simulink model "ltao_e2e"  (R2022b)
settings: Solver=FixedStepDiscrete  StartTime=0.0  StopTime=30  FixedStep=FEM_Ts  MaxStep=FEM_Ts  RelTol=1e-2
InitFcn:
  | %
  | % Initialization callback function
  | %
  | 
  | try
  |    fprintf('\nGMT IMS version (%s)!\n',simulink_fname );
  | 
  |    % Get Simulink model directory
  |    [filepath,name,ext] = fileparts(which(bdroot));
  | 
  |    if ~strcmp(filepath,pwd)
  |       fprintf('\nChanging current directory to \n %s \n',filepath);
  |       cd(filepath);
  |    end
  | 
  |    %
  |  if(osim.bpless_wl)
  |     fprintf('Generating bumpless wind load time series\n');
  |  end
  | catch
  |    warning('Running the InitFcn from puSimulate script');
  | end
values from neighbouring files (symbols this model uses):
  asm_kl_dist = 0*asm_kl_dist    [load_ltao_e2e.m]
  asm_ssG = XiKL' * asm_ssG * XiKL    [load_ltao_e2e.m]
  Cpi_d = eye(n_Zmodes)* c2d(st.asm.fpi, Ts, c2d_opts)    [evalM2asm_modal.m]    (also in load_ltao_e2e.m = c2d(st.asm.fpi, FEM_Ts, c2d_opts))
  fao_d = c2d(st.glao.fao, st.glao.T, c2d_opts)    [evalM2asm_modal.m]    (also in load_ltao_e2e.m = c2d(st.ltao.fao, FEM_Ts, c2d_opts))
  fao_d4k = c2d(st.ltao.fao, 1/4e3, c2d_opts)    [evalM2asm_modal.m]    (also in load_ltao_e2e.m = c2d(st.ltao.fao, FEM_Ts, c2d_opts))
  FEM_Ts = 1/8e3    (= 0.000125)    [load_ltao_e2e.m]
  fes = c2d(tf((fc_es^2)*4*(pi^2),[1, 2*0.8*fc_es*2*pi, (fc_es^2)*4*(pi^2)]),     st.ltao.T,c2d_opts)    [load_ltao_e2e.m]
  flag_1stOdyn_d = tf(c2d(flag(2,1), Ts, c2d_opts))    [evalM2asm_modal.m]    (also in load_ltao_e2e.m = tf(c2d(flag(2,1),FEM_Ts,c2d_opts)))
  flag_2ndOdyn_d = tf(c2d(flag(3,1), Ts, c2d_opts))    [evalM2asm_modal.m]    (also in load_ltao_e2e.m = tf(c2d(flag(3,1),FEM_Ts,c2d_opts)))
  fm2off = c2d(f_ct_m2off, st.ltao.T,c2d_opts)    [load_ltao_e2e.m]
  fpre_d = tf(c2d(st.asm.fpre, Ts, c2d_opts))    [evalM2asm_modal.m]    (also in load_ltao_e2e.m = tf(c2d(fpre,FEM_Ts,c2d_opts)))
  gtt2mnt = eye(2)/(rbm2gtt * Hk_mnt_m1m2)    [load_ltao_e2e.m]
  Hk_mnt_m1m2 = Cm1m2*pinv(Cmnt)    [load_ltao_e2e.m]
  Hpd_d = eye(n_Zmodes)* c2d(st.asm.fpd, Ts, c2d_opts)    [evalM2asm_modal.m]    (also in load_ltao_e2e.m = c2d(st.asm.fpd, FEM_Ts, 'Tustin'))
  K_asm_2_m2p = K_m2p / K_m2p6F_2_asmRB    [load_ltao_e2e.m]
  K_m2p = gainMatrix(out_m2p_mc,in_m2p_mc) -gainMatrix(out_m2p_mc,in_m2p_m2)          - gainMatrix(out_m2p_m2,in_m2p_mc) +gainMatrix(out_m2p_m2,in_m2p_m2)    [load_ltao_e2e.m]
  K_m2p6F_2_asmRB = gainMatrix(out_asm_RB,in_m2p_mc) - gainMatrix(out_asm_RB,in_m2p_m2)    [load_ltao_e2e.m]
  K_m2p_2_asm = K_m2p6F_2_asmRB/ K_m2p    [load_ltao_e2e.m]
  K_m2p_2_es = gainMatrix(out_m2es,in_m2p_mc)-gainMatrix(out_m2es,in_m2p_m2)    [load_ltao_e2e.m]
  Kasmoff = K_asm_2_m2p *         [Kasmoff_{1},Kasmoff_{2},Kasmoff_{3},Kasmoff_{4},         Kasmoff_{5},Kasmoff_{6},Kasmoff_{7}]    [load_ltao_e2e.m]
  Ki_m2off = 1.3    [load_ltao_e2e.m]
  Km1rbm_es = (KhpF2es/KhpF2m1rbm)    [load_ltao_e2e.m]
  Ks = cell(7,1)    [load_ltao_e2e.m]
  m1_rbm_dist = zeros(42,1)    [load_ltao_e2e.m]
  m2_rbm_dist = 0*m2_rbm_dist    [load_ltao_e2e.m]
  m2_rbm_offset = 0*m2_rbm_offset    [load_ltao_e2e.m]
  PG = zeros(length(om2),6)    [evalM2asm_modal.m]    (also in load_ltao_e2e.m)
  phiB = inputs2ModalF(mode_ind_vec,indDesInputs) * KinputT    [load_ltao_e2e.m]
  phiC = KoutputT * modalDisp2Outputs(indDesOutputs,mode_ind_vec)    [load_ltao_e2e.m]
  Psi_ss = KoutputT *gainMatrix(indDesOutputs,indDesInputs)* KinputT - K_ss    [load_ltao_e2e.m]
  Rm2es = pinv(K_asm_2_es, 1e-2)    [load_ltao_e2e.m]
  segPTT2asmCMD = cell(7,1)    [load_ltao_e2e.m]
  st = getcontrol_asm()    [evalM2asm_modal.m]    (also in load_ltao_e2e.m)
  T_pos2e = (K_m2p_2_es / K_m2p)    [load_ltao_e2e.m]
undefined symbols (not defined in the file or in its folder): a, az, az_ff_en, b, c, D_seg_piston, D_seg_tt, DiscIntNeverNeededParam, el, fem, gir, m1sys, m2pos, magnitude, mount, osim, rbm2gtt, Rm1es, sm, VC_modal_stiff
libraries: ims_block_library x7, simulink x2
(part 3 of 3)

== system ltao_e2e/M2 Control/ASMmodal_Control/ASM_inner_loop_controller_S7 ==
  ASM_cmd : Inport
  ASM_FB : Inport  Port=2
  ASM Input filter : DiscreteTransferFcn  Numerator=fpre_d.num{1}  Denominator=fpre_d.den{1}  SampleTime=fpre_d.Ts
  ASM PI controller : DiscreteTransferFcn  Numerator=Cpi_d.num{1}  Denominator=Cpi_d.den{1}  SampleTime=Cpi_d.Ts
  Kb : Gain  Gain=st.asm.Kb
  Kd : Gain  Gain=st.asm.Kd
  Km : Gain  Gain=st.asm.Km
  Ks : Gain  Gain=Ks{7}  Multiplication=Matrix(K*u)
  Numerical differentiation : DiscreteTransferFcn  Numerator=Hpd_d.num{1}  Denominator=Hpd_d.den{1}  SampleTime=Hpd_d.Ts
  Sum1 : Sum  Inputs=|+-
  Sum2 : Sum
  Sum3 : Sum  Inputs=|+-
  Sum4 : Sum  Inputs=++|
  Sum5 : Sum
  m2_asm_ff_en : Gain  Gain=osim.m2_asm_ff_en
  s*fpre (DT version) : DiscreteTransferFcn  Numerator=flag_1stOdyn_d.num{1}  Denominator=flag_1stOdyn_d.den{1}  SampleTime=flag_1stOdyn_d.Ts
  s^2*fpre (DT version) : DiscreteTransferFcn  Numerator=flag_2ndOdyn_d.num{1}  Denominator=flag_2ndOdyn_d.den{1}  SampleTime=flag_2ndOdyn_d.Ts
  ASM_modalF : Outport  VectorParamsAs1DForOutWhenUnconnected=off
  Mag_modal_vel : Outport  Port=2  VectorParamsAs1DForOutWhenUnconnected=off
  wires:
  m2_asm_ff_en/1 -> Sum4/1
  s*fpre (DT version)/1 -> Kb/1
  ASM PI controller/1 -> Sum3/1
  Sum3/1 -> Sum4/2
  Km/1 -> Sum5/1
  Kb/1 -> Sum5/2
  Ks/1 -> Sum2/2
  s^2*fpre (DT version)/1 -> Km/1
  Kd/1 -> Sum3/2
  Sum5/1 -> Sum2/1
  ASM_FB/1 -> Numerical differentiation/1, Sum1/2
  ASM_cmd/1 -> s^2*fpre (DT version)/1, s*fpre (DT version)/1, ASM Input filter/1
  Sum1/1 -> ASM PI controller/1
  Sum4/1 -> ASM_modalF/1
  Sum2/1 -> m2_asm_ff_en/1
  Numerical differentiation/1 -> Mag_modal_vel/1, Kd/1
  ASM Input filter/1 -> Ks/1, Sum1/1

== system ltao_e2e/M2 Control/M2 ES Controller/segPTT2asmCMD ==
  segTTP : Inport
  Mux : Mux  Inputs=7
  PTT2ASM_S1 : Gain  Gain=segPTT2asmCMD{1}  Multiplication=Matrix(K*u)
  PTT2ASM_S2 : Gain  Gain=segPTT2asmCMD{2}  Multiplication=Matrix(K*u)
  PTT2ASM_S3 : Gain  Gain=segPTT2asmCMD{3}  Multiplication=Matrix(K*u)
  PTT2ASM_S4 : Gain  Gain=segPTT2asmCMD{4}  Multiplication=Matrix(K*u)
  PTT2ASM_S5 : Gain  Gain=segPTT2asmCMD{5}  Multiplication=Matrix(K*u)
  PTT2ASM_S6 : Gain  Gain=segPTT2asmCMD{6}  Multiplication=Matrix(K*u)
  PTT2ASM_S7 : Gain  Gain=segPTT2asmCMD{7}  Multiplication=Matrix(K*u)
  Selector_S1 : Selector  InputPortWidth=21  IndexOptions=Index vector (dialog)  Indices=1:7:21  OutputSizes=1
  Selector_S2 : Selector  InputPortWidth=21  IndexOptions=Index vector (dialog)  Indices=2:7:21  OutputSizes=1
  Selector_S3 : Selector  InputPortWidth=21  IndexOptions=Index vector (dialog)  Indices=3:7:21  OutputSizes=1
  Selector_S4 : Selector  InputPortWidth=21  IndexOptions=Index vector (dialog)  Indices=4:7:21  OutputSizes=1
  Selector_S5 : Selector  InputPortWidth=21  IndexOptions=Index vector (dialog)  Indices=5:7:21  OutputSizes=1
  Selector_S6 : Selector  InputPortWidth=21  IndexOptions=Index vector (dialog)  Indices=6:7:21  OutputSizes=1
  Selector_S7 : Selector  InputPortWidth=21  IndexOptions=Index vector (dialog)  Indices=7:7:21  OutputSizes=1
  ASM_KL012_CMD : Outport
  wires:
  Mux/1 -> ASM_KL012_CMD/1
  PTT2ASM_S7/1 -> Mux/7
  PTT2ASM_S6/1 -> Mux/6
  PTT2ASM_S5/1 -> Mux/5
  PTT2ASM_S3/1 -> Mux/3
  PTT2ASM_S4/1 -> Mux/4
  PTT2ASM_S2/1 -> Mux/2
  Selector_S4/1 -> PTT2ASM_S4/1
  PTT2ASM_S1/1 -> Mux/1
  Selector_S7/1 -> PTT2ASM_S7/1
  Selector_S6/1 -> PTT2ASM_S6/1
  Selector_S3/1 -> PTT2ASM_S3/1
  Selector_S2/1 -> PTT2ASM_S2/1
  Selector_S1/1 -> PTT2ASM_S1/1
  Selector_S5/1 -> PTT2ASM_S5/1
  segTTP/1 -> Selector_S7/1, Selector_S6/1, Selector_S5/1, Selector_S4/1, Selector_S3/1, Selector_S2/1, Selector_S1/1

== system ltao_e2e/Mount_Drv_PDR2021_linear/AZ DT Lugre Fr model/g(v) ==
  v : Inport
  Enable : EnablePort
  Constant : Constant  Value=0
  gs : Subsystem
  g : Outport  VectorParamsAs1DForOutWhenUnconnected=off
  wires:
  gs/1(gs(v)) -> g/1
  v/1 -> gs/1(v)
  Constant/1 -> gs/Enable

== system ltao_e2e/Mount_Drv_PDR2021_linear/AZ DT Lugre Fr model/v2z ==
  v : Inport
  g(v) : Inport  Port=2
  z : Inport  Port=3
  Enable : EnablePort
  Abs : Abs  SaturateOnIntegerOverflow=off
  Divide : Product  Inputs=*/*
  Sum : Sum  Inputs=|+-
  dz : Outport  VectorParamsAs1DForOutWhenUnconnected=off
  wires:
  Abs/1 -> Divide/1
  Divide/1 -> Sum/2
  v/1 -> Sum/1, Abs/1
  Sum/1 -> dz/1
  g(v)/1 -> Divide/2
  z/1 -> Divide/3

== system ltao_e2e/Mount_Drv_PDR2021_linear/EL DT Lugre Fr model/g(v) ==
  v : Inport
  Enable : EnablePort
  Constant : Constant  Value=0
  Sum : Sum  Inputs=|++
  gc : Constant  Value=frParStruct.Tc/frParStruct.sigm0
  gs : Subsystem
  g : Outport  VectorParamsAs1DForOutWhenUnconnected=off
  wires:
  Sum/1 -> g/1
  v/1 -> gs/1(v)
  gs/1(gs(v)) -> Sum/1
  gc/1 -> Sum/2
  Constant/1 -> gs/Enable

== system ltao_e2e/Mount_Drv_PDR2021_linear/EL DT Lugre Fr model/v2z ==
  v : Inport
  g(v) : Inport  Port=2
  z : Inport  Port=3
  Enable : EnablePort
  Abs : Abs  SaturateOnIntegerOverflow=off
  Divide : Product  Inputs=*/*
  Sum : Sum  Inputs=|+-
  dz : Outport  VectorParamsAs1DForOutWhenUnconnected=off
  wires:
  Abs/1 -> Divide/1
  Divide/1 -> Sum/2
  v/1 -> Sum/1, Abs/1
  Sum/1 -> dz/1
  g(v)/1 -> Divide/2
  z/1 -> Divide/3

== system ltao_e2e/Mount_Drv_PDR2021_linear/GIR DT Lugre Fr model/g(v) ==
  v : Inport
  Constant : Constant  Value=0
  Sum : Sum  Inputs=|++
  gc : Constant  Value=frParStruct.Tc/frParStruct.sigm0
  gs : Subsystem
  g : Outport  VectorParamsAs1DForOutWhenUnconnected=off
  wires:
  Sum/1 -> g/1
  v/1 -> gs/1(v)
  gs/1(gs(v)) -> Sum/1
  gc/1 -> Sum/2
  Constant/1 -> gs/Enable

== system ltao_e2e/Mount_Drv_PDR2021_linear/GIR DT Lugre Fr model/v2z ==
  v : Inport
  g(v) : Inport  Port=2
  z : Inport  Port=3
  Abs : Abs  SaturateOnIntegerOverflow=off
  Divide : Product  Inputs=*/*
  Sum : Sum  Inputs=|+-
  dz : Outport  VectorParamsAs1DForOutWhenUnconnected=off
  wires:
  Abs/1 -> Divide/1
  Divide/1 -> Sum/2
  v/1 -> Sum/1, Abs/1
  Sum/1 -> dz/1
  g(v)/1 -> Divide/2
  z/1 -> Divide/3

== system ltao_e2e/Mount_Drv_PDR2021_linear/Parasitic torques model /AZ_Parasitic_Torque ==
  Drive_Pos : Inport
  Drive_Torque : Inport  Port=2
  Cogging : Lookup_n-D  NumberOfTableDimensions=1  LookupTableObject=F_ripple  BreakpointsForDimension1=ParasiticModelStruc.Pos  Table=ParasiticModelStruc.oCog.Amp  InternalRulePriority=Speed  RndMeth=Simplest
  Constant : Constant  Value=0.1869
  Divide : Product  Inputs=**
  EMF Distortion : Lookup_n-D  NumberOfTableDimensions=1  LookupTableObject=F_ripple  BreakpointsForDimension1=ParasiticModelStruc.Pos  Table=ParasiticModelStruc.oEmf.Amp  InternalRulePriority=Speed  RndMeth=Simplest
  Gain : Gain  Gain=1/ParasiticModelStruc.R
  Gain1 : Gain  Gain=1/250
  Gain2 : Gain  Gain=1/ParasiticModelStruc.N_Segm
  Mod : Math  Operator=rem  SignedPower=on
  Mod1 : Math  Operator=rem  SignedPower=on
  Radius : Gain  Gain=ParasiticModelStruc.R
  Sum1 : Sum
  Sum2 : Sum
  Parasitic_Torque : Outport  VectorParamsAs1DForOutWhenUnconnected=off
  wires:
  Divide/1 -> Sum1/1
  Gain1/1 -> Gain2/1  "I_rms"
  Mod1/1 -> EMF Distortion/1, Cogging/1
  Cogging/1 -> Sum1/2
  Radius/1 -> Mod/1  "driven  distance"
  Drive_Torque/1 -> Gain/1
  Gain/1 -> Gain1/1  "Force"
  EMF Distortion/1 -> Divide/2
  Sum2/1 -> Mod1/1
  Mod/1 -> Sum2/1
  Gain2/1 -> Divide/1  "I_rms pro Segment"
  Constant/1 -> Mod/2, Sum2/2, Mod1/2
  Drive_Pos/1 -> Radius/1  "Drive Position"
  Sum1/1 -> Parasitic_Torque/1

== system ltao_e2e/Mount_Drv_PDR2021_linear/Parasitic torques model /EL_Parasitic_Torque ==
  Drive_Pos : Inport
  Drive_Torque : Inport  Port=2
  Cogging : Lookup_n-D  NumberOfTableDimensions=1  LookupTableObject=F_ripple  BreakpointsForDimension1=ParasiticModelStruc.Pos  Table=ParasiticModelStruc.oCog.Amp  InternalRulePriority=Speed  RndMeth=Simplest
  Constant : Constant  Value=0.1869
  Divide : Product  Inputs=**
  EMF Distortion : Lookup_n-D  NumberOfTableDimensions=1  LookupTableObject=F_ripple  BreakpointsForDimension1=ParasiticModelStruc.Pos  Table=ParasiticModelStruc.oEmf.Amp  InternalRulePriority=Speed  RndMeth=Simplest
  Gain : Gain  Gain=1/ParasiticModelStruc.R
  Gain1 : Gain  Gain=1/250
  Gain2 : Gain  Gain=1/ParasiticModelStruc.N_Segm
  Mod : Math  Operator=rem  SignedPower=on
  Mod1 : Math  Operator=rem  SignedPower=on
  Radius : Gain  Gain=ParasiticModelStruc.R
  Sum1 : Sum
  Sum2 : Sum
  Parasitic_Torque : Outport  VectorParamsAs1DForOutWhenUnconnected=off
  wires:
  Sum1/1 -> Parasitic_Torque/1
  Drive_Torque/1 -> Gain/1
  EMF Distortion/1 -> Divide/2
  Drive_Pos/1 -> Radius/1  "Drive Position"
  Gain1/1 -> Gain2/1  "I_rms"
  Gain2/1 -> Divide/1  "I_rms pro Segment"
  Gain/1 -> Gain1/1  "Force"
  Mod/1 -> Sum2/1
  Cogging/1 -> Sum1/2
  Radius/1 -> Mod/1  "driven  distance"
  Sum2/1 -> Mod1/1
  Mod1/1 -> EMF Distortion/1, Cogging/1
  Divide/1 -> Sum1/1
  Constant/1 -> Mod/2, Sum2/2, Mod1/2

== system ltao_e2e/Mount_Drv_PDR2021_linear/Parasitic torques model /GIR_Parasitic_Torque ==
  note: EMF Torque Model
  note: Cogging Torque Model
  Drive_Pos : Inport
  Drive_Torque : Inport  Port=2
  CogAmp : Constant  Value=ParasiticModelStruc.oCog.amp
  CogSpatFreq : Constant  Value=ParasiticModelStruc.oCog.sfr
  Product : Product
  Product1 : Product  RndMeth=Zero
  Product2 : Product  Inputs=3  RndMeth=Zero
  Product3 : Product  RndMeth=Zero
  Product4 : Product  RndMeth=Zero
  RippleAmpFactor : Constant  Value=ParasiticModelStruc.oEmf.ampFact
  RippleSpatFreq : Constant  Value=ParasiticModelStruc.oEmf.sfr
  Sign : Signum
  Sum : Sum  Inputs=|++
  Sum1 : Sum  Inputs=++|
  ToPretension : Constant  Value=T_pretension
  Trigonometric Function : Trigonometry
  Trigonometric Function1 : Trigonometry
  Parasitic_Torque : Outport  VectorParamsAs1DForOutWhenUnconnected=off
  wires:
  RippleAmpFactor/1 -> Product2/2
  Product1/1 -> Trigonometric Function/1
  RippleSpatFreq/1 -> Product1/2
  Product3/1 -> Trigonometric Function1/1
  Trigonometric Function1/1 -> Product4/1
  CogSpatFreq/1 -> Product3/2
  Drive_Pos/1 -> Product3/1, Product1/1  "Drive Position"
  CogAmp/1 -> Product4/2
  Product4/1 -> Sum/2
  Product2/1 -> Sum/1
  Sum/1 -> Parasitic_Torque/1
  Trigonometric Function/1 -> Product2/3
  Sum1/1 -> Product2/1
  Drive_Torque/1 -> Sign/1, Sum1/2  "Drive Torque (Nm)"
  Sign/1 -> Product/2
  ToPretension/1 -> Product/1
  Product/1 -> Sum1/1

== system ltao_e2e/Mount_Drv_PDR2021_linear/Parasitic torques model /Subsystem ==
  Az Pos : Inport
  Az To : Inport  Port=2
  El Pos : Inport  Port=3
  El To : Inport  Port=4
  Gir Pos : Inport  Port=5
  Gir To : Inport  Port=6
  Constant2 : Constant
  Demux1 : Demux  Outputs=3
  Mux1 : Mux  Inputs=3
  Mux7 : Mux  Inputs=3
  Parasitic Torques : Subsystem
  Out1 : Outport  VectorParamsAs1DForOutWhenUnconnected=off
  Out2 : Outport  Port=2  VectorParamsAs1DForOutWhenUnconnected=off
  Out3 : Outport  Port=3  VectorParamsAs1DForOutWhenUnconnected=off
  wires:
  Demux1/1 -> Out1/1
  Demux1/2 -> Out2/1
  Gir Pos/1 -> Mux7/3
  Demux1/3 -> Out3/1
  Az Pos/1 -> Mux7/1
  Mux7/1 -> Parasitic Torques/2(MotPos)
  Mux1/1 -> Parasitic Torques/1(MotTo)
  Constant2/1 -> Parasitic Torques/Enable
  El Pos/1 -> Mux7/2
  Parasitic Torques/1(ParasiticTo) -> Demux1/1
  Az To/1 -> Mux1/1
  El To/1 -> Mux1/2
  Gir To/1 -> Mux1/3

== system ltao_e2e/Telescope model/Structural Dynamics GMT/FEM_SS ==
  note: 2nd order form simulation
  In : Inport
  Mount vel gnd : Terminator  Commented=on
  Sum2 : Sum  Inputs=+++
  Sum3 : Sum  Inputs=+++
  Unit Delay : UnitDelay  SampleTime=FEM_Ts  HasFrameUpgradeWarning=on
  Unit Delay1 : UnitDelay  SampleTime=FEM_Ts  HasFrameUpgradeWarning=on
  gamma1 : Gain  Gain=PG(:,3)
  gamma2 : Gain  Gain=PG(:,6)
  phi11 : Gain  Gain=PG(:,1)
  phi12 : Gain  Gain=PG(:,2)
  phi21 : Gain  Gain=PG(:,4)
  phi22 : Gain  Gain=PG(:,5)
  phiB : Gain  Gain=phiB  Multiplication=Matrix(K*u) (u vector)
  phiC : Gain  Gain=phiC  Multiplication=Matrix(K*u) (u vector)
  phiCv : Gain  Gain=phiC(1:14,:)  Multiplication=Matrix(K*u) (u vector)
  pos : Outport  VectorParamsAs1DForOutWhenUnconnected=off
  mount_vel : Outport  Port=2  VectorParamsAs1DForOutWhenUnconnected=off
  wires:
  phiCv/1 -> Mount vel gnd/1, mount_vel/1
  In/1 -> phiB/1
  phiC/1 -> pos/1
  phiB/1 -> gamma1/1, gamma2/1
  Unit Delay1/1 -> phi22/1, phi12/1, phiCv/1
  phi11/1 -> Sum3/3
  gamma1/1 -> Sum3/1
  phi22/1 -> Sum2/1
  phi21/1 -> Sum2/2
  gamma2/1 -> Sum2/3
  Sum3/1 -> Unit Delay/1
  Sum2/1 -> Unit Delay1/1
  phi12/1 -> Sum3/2
  Unit Delay/1 -> phiC/1, phi21/1, phi11/1

== system ltao_e2e/Telescope model/Structural Dynamics GMT_/FEM_SS ==
  note: 2nd order form simulation
  In : Inport
  Mount vel gnd : Terminator  Commented=on
  Sum2 : Sum  Inputs=+++
  Sum3 : Sum  Inputs=+++
  Unit Delay : UnitDelay  SampleTime=FEM_Ts  HasFrameUpgradeWarning=on
  Unit Delay1 : UnitDelay  SampleTime=FEM_Ts  HasFrameUpgradeWarning=on
  gamma1 : Gain  Gain=PG(:,3)
  gamma2 : Gain  Gain=PG(:,6)
  phi11 : Gain  Gain=PG(:,1)
  phi12 : Gain  Gain=PG(:,2)
  phi21 : Gain  Gain=PG(:,4)
  phi22 : Gain  Gain=PG(:,5)
  phiB : Gain  Gain=phiB  Multiplication=Matrix(K*u) (u vector)
  phiC : Gain  Gain=phiC  Multiplication=Matrix(K*u) (u vector)
  phiCv : Gain  Gain=phiC(1:14,:)  Multiplication=Matrix(K*u) (u vector)
  pos : Outport  VectorParamsAs1DForOutWhenUnconnected=off
  mount_vel : Outport  Port=2  VectorParamsAs1DForOutWhenUnconnected=off
  wires:
  Unit Delay/1 -> phi11/1, phi21/1, phiC/1
  phi12/1 -> Sum3/2
  Sum2/1 -> Unit Delay1/1
  Sum3/1 -> Unit Delay/1
  gamma2/1 -> Sum2/3
  phi21/1 -> Sum2/2
  phi22/1 -> Sum2/1
  gamma1/1 -> Sum3/1
  phi11/1 -> Sum3/3
  Unit Delay1/1 -> phiCv/1, phi12/1, phi22/1
  phiB/1 -> gamma2/1, gamma1/1
  phiC/1 -> pos/1
  In/1 -> phiB/1
  phiCv/1 -> mount_vel/1, Mount vel gnd/1

== system ltao_e2e/M2 Control/ASMmodal_Control/ASM_inner_loop_controller_S2/Pre shape + FF terms ==
  cmd : Inport  PortDimensions=length(VC_modal_stiff{1})
  " 1" : Constant  Commented=on  Value=sm.tSF
  " 2" : Constant  Commented=on  Value=sm.d1SF
  " 3" : Constant  Commented=on  Value=sm.d2SF
  " 4" : Constant  Commented=on  Value=sm.d3SF
  " 5" : Constant  Commented=on  Value=sm.TCmd
  Clock : Clock  Commented=on
  Cmd Shaping Filter : Subsystem
  Command Shaping Filter : MATLAB Function  Commented=on  TreatAsAtomicUnit=on  SystemSampleTime=FEM_Ts
  Memory : Memory  Commented=on  InheritSampleTime=on
  Mux : Mux  Commented=on  Inputs=2
  RTout : RateTransition  Commented=on  OutPortSampleTime=FEM_Ts
  RTout_CMdOld : RateTransition  Commented=on  OutPortSampleTime=FEM_Ts
  Scope : Scope  Commented=on
  Selector : Selector  Commented=on  InputPortWidth=66  IndexOptions=Index vector (dialog)  Indices=[1 2 4]  OutputSizes=1
  Selector1 : Selector  Commented=on  InputPortWidth=66  IndexOptions=Index vector (dialog)  Indices=[1 2 4]  OutputSizes=1
  SFdd : Outport  PortDimensions=length(VC_modal_stiff{1})  VectorParamsAs1DForOutWhenUnconnected=off
  SFd : Outport  Port=2  PortDimensions=length(VC_modal_stiff{1})  VectorParamsAs1DForOutWhenUnconnected=off
  SF : Outport  Port=3  PortDimensions=length(VC_modal_stiff{1})  VectorParamsAs1DForOutWhenUnconnected=off
  wires:
  " 4"/1 -> Command Shaping Filter/8(d3SF)
  Clock/1 -> Command Shaping Filter/3(t)
  cmd/1 -> RTout/1, Memory/1, Cmd Shaping Filter/1(cmd)
  " 1"/1 -> Command Shaping Filter/5(tSF)
  " 3"/1 -> Command Shaping Filter/7(d2SF)
  " 2"/1 -> Command Shaping Filter/6(d1SF)
  Memory/1 -> RTout_CMdOld/1
  RTout/1 -> Command Shaping Filter/2(cmd)
  RTout_CMdOld/1 -> Command Shaping Filter/1(cmdOld)
  Selector/1 -> Mux/1
  Selector1/1 -> Mux/2
  Mux/1 -> Scope/1
  " 5"/1 -> Command Shaping Filter/4(Tcmd)
  Cmd Shaping Filter/3(SF) -> SF/1
  Cmd Shaping Filter/1(SFdd) -> SFdd/1, Selector/1
  Cmd Shaping Filter/2(SFd) -> SFd/1
  Command Shaping Filter/1(cmdSFdd) -> Selector1/1

== system ltao_e2e/Mount_Drv_PDR2021_linear/AZ DT Lugre Fr model/g(v)/gs ==
  v : Inport
  Enable : EnablePort
  Divide : Product  Inputs=**
  Gain : Gain  Gain=1/frParStruct.vs
  Math Function : Math  SignedPower=on
  Math Function1 : Math  Operator=magnitude^2  SignedPower=on
  Sum : Sum  Inputs=|++
  Unary Minus : UnaryMinus
  gc : Constant  Value=frParStruct.Tc/frParStruct.sigm0
  gs : Constant  Value=(frParStruct.Ts-frParStruct.Tc)/frParStruct.sigm0
  gs(v) : Outport  VectorParamsAs1DForOutWhenUnconnected=off
  wires:
  Math Function/1 -> Divide/1
  gs/1 -> Divide/2
  Math Function1/1 -> Unary Minus/1
  Unary Minus/1 -> Math Function/1
  Gain/1 -> Math Function1/1
  v/1 -> Gain/1
  gc/1 -> Sum/2
  Divide/1 -> Sum/1
  Sum/1 -> gs(v)/1

== system ltao_e2e/Mount_Drv_PDR2021_linear/EL DT Lugre Fr model/g(v)/gs ==
  v : Inport
  Enable : EnablePort
  Divide : Product  Inputs=**
  Gain : Gain  Gain=1/frParStruct.vs
  Math Function : Math  SignedPower=on
  Math Function1 : Math  Operator=magnitude^2  SignedPower=on
  Unary Minus : UnaryMinus
  gs : Constant  Value=(frParStruct.Ts-frParStruct.Tc)/frParStruct.sigm0
  gs(v) : Outport  VectorParamsAs1DForOutWhenUnconnected=off
  wires:
  Math Function/1 -> Divide/1
  gs/1 -> Divide/2
  Math Function1/1 -> Unary Minus/1
  Unary Minus/1 -> Math Function/1
  Gain/1 -> Math Function1/1
  v/1 -> Gain/1
  Divide/1 -> gs(v)/1

== system ltao_e2e/Mount_Drv_PDR2021_linear/GIR DT Lugre Fr model/g(v)/gs ==
  v : Inport
  Enable : EnablePort
  Divide : Product  Inputs=**
  Gain : Gain  Gain=1/frParStruct.vs
  Math Function : Math  SignedPower=on
  Math Function1 : Math  Operator=magnitude^2  SignedPower=on
  Unary Minus : UnaryMinus
  gs : Constant  Value=(frParStruct.Ts-frParStruct.Tc)/frParStruct.sigm0
  gs(v) : Outport  VectorParamsAs1DForOutWhenUnconnected=off
  wires:
  Math Function/1 -> Divide/1
  gs/1 -> Divide/2
  Math Function1/1 -> Unary Minus/1
  Unary Minus/1 -> Math Function/1
  Gain/1 -> Math Function1/1
  v/1 -> Gain/1
  Divide/1 -> gs(v)/1

== system ltao_e2e/Mount_Drv_PDR2021_linear/Parasitic torques model /Subsystem/Parasitic Torques ==
  MotTo : Inport
  MotPos : Inport  Port=2
  Enable : EnablePort
  Demux1 : Demux  Outputs=2
  Demux2 : Demux  Outputs=2
  Demux3 : Demux  Outputs=2
  Mux2 : Mux  Inputs=2
  Mux3 : Mux  Inputs=3
  Parasitic AZ : Subsystem  mask{Pos=az.oParasitic.Pos, Amp_Cog=az.oParasitic.oCog.Amp, Amp_EMF=az.oParasitic.oEmf.Amp, R=az.oParasitic.R, N_Segm=az.oParasitic.N_Segm}
  Parasitic EL : Subsystem  mask{Pos=el.oParasitic.Pos, Amp_Cog=el.oParasitic.oCog.Amp, Amp_EMF=el.oParasitic.oEmf.Amp, R=el.oParasitic.R, N_Segm=el.oParasitic.N_Segm}
  Parasitic GIR : Subsystem  mask{cog_sfr=gir.oParasitic.oCog.sfr, cog_amp=gir.oParasitic.oCog.amp, emf_sfr=gir.oParasitic.oEmf.sfr, emf_ampFact=gir.oParasitic.oEmf.ampFact, T_pretension=gir.T_pretension}
  Sel : Selector  InputPortWidth=6  IndexOptions=Index vector (dialog)  Indices=[1 4]  OutputSizes=1
  Sel1 : Selector  InputPortWidth=6  IndexOptions=Index vector (dialog)  Indices=[2 5]  OutputSizes=1
  Sel2 : Selector  InputPortWidth=6  IndexOptions=Index vector (dialog)  Indices=[3 6]  OutputSizes=1
  ParasiticTo : Outport
  wires:
  Mux3/1 -> ParasiticTo/1
  Mux2/1 -> Sel/1, Sel2/1, Sel1/1
  MotTo/1 -> Mux2/1
  MotPos/1 -> Mux2/2
  Sel/1 -> Demux3/1
  Demux3/2 -> Parasitic AZ/2(MotPos)
  Parasitic AZ/1(To) -> Mux3/1
  Sel1/1 -> Demux1/1
  Demux1/2 -> Parasitic EL/2(MotPos)
  Parasitic EL/1(To) -> Mux3/2
  Demux2/1 -> Parasitic GIR/1(MotTo)
  Demux2/2 -> Parasitic GIR/2(MotPos)
  Sel2/1 -> Demux2/1
  Demux3/1 -> Parasitic AZ/1(MotTo)
  Demux1/1 -> Parasitic EL/1(MotTo)
  Parasitic GIR/1(To) -> Mux3/3

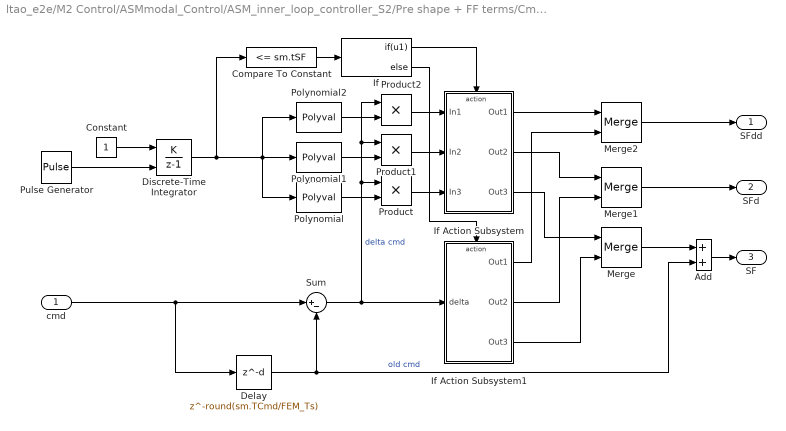
== system ltao_e2e/M2 Control/ASMmodal_Control/ASM_inner_loop_controller_S2/Pre shape + FF terms/Cmd Shaping Filter ==
  cmd : Inport
  Add : Sum
  Compare To Constant : simulink/Logic and Bit Operations/Compare To Constant  relop=<=  const=sm.tSF  OutDataTypeStr=boolean
  Constant : Constant
  Delay : Delay  DelayLength=round(sm.TCmd/FEM_Ts)
  Discrete-Time Integrator : DiscreteIntegrator  IntegratorMethod=Accumulation: Forward Euler  gainval=FEM_Ts  ExternalReset=rising  SampleTime=FEM_Ts  ICPrevOutput=DiscIntNeverNeededParam  ICPrevScaledInput=DiscIntNeverNeededParam
  If : If  IfExpression=u1
  If Action Subsystem : Subsystem  TreatAsAtomicUnit=on
  If Action Subsystem1 : Subsystem  TreatAsAtomicUnit=on
  Merge : Merge
  Merge1 : Merge
  Merge2 : Merge
  Polynomial : Polyval  Coefs=[sm.d3SF/20, sm.d2SF/12, sm.d1SF/6, 0, 0, 0]
  Polynomial1 : Polyval  Coefs=[5*sm.d3SF/20, 4*sm.d2SF/12, 3*sm.d1SF/6, 0, 0]
  Polynomial2 : Polyval  Coefs=[20*sm.d3SF/20, 12*sm.d2SF/12, 6*sm.d1SF/6, 0]
  Product : Product
  Product1 : Product
  Product2 : Product
  Pulse Generator : DiscretePulseGenerator  Period=round(sm.TCmd/FEM_Ts)  SampleTime=FEM_Ts
  Sum : Sum  Inputs=|+-
  SFdd : Outport  VectorParamsAs1DForOutWhenUnconnected=off
  SFd : Outport  Port=2  VectorParamsAs1DForOutWhenUnconnected=off
  SF : Outport  Port=3  VectorParamsAs1DForOutWhenUnconnected=off
  wires:
  Discrete-Time Integrator/1 -> Compare To Constant/1, Polynomial2/1, Polynomial/1, Polynomial1/1
  Constant/1 -> Discrete-Time Integrator/1
  Polynomial1/1 -> Product1/2
  Polynomial/1 -> Product/2
  Polynomial2/1 -> Product2/2
  Sum/1 -> If Action Subsystem1/1(delta), Product2/1, Product1/1, Product/1  "delta cmd"
  Add/1 -> SF/1
  Compare To Constant/1 -> If/1
  Product/1 -> If Action Subsystem/3(In3)
  Product1/1 -> If Action Subsystem/2(In2)
  Product2/1 -> If Action Subsystem/1(In1)
  Merge1/1 -> SFd/1
  Merge/1 -> Add/1
  Delay/1 -> Sum/2, Add/2  "old cmd"
  If/1 -> If Action Subsystem/Action
  If/2 -> If Action Subsystem1/Action
  Merge2/1 -> SFdd/1
  If Action Subsystem/1(Out1) -> Merge2/1
  If Action Subsystem1/1(Out1) -> Merge2/2
  If Action Subsystem/2(Out2) -> Merge1/1
  If Action Subsystem/3(Out3) -> Merge/1
  If Action Subsystem1/2(Out2) -> Merge1/2
  If Action Subsystem1/3(Out3) -> Merge/2
  Pulse Generator/1 -> Discrete-Time Integrator/2
  cmd/1 -> Delay/1, Sum/1

== system ltao_e2e/Mount_Drv_PDR2021_linear/Parasitic torques model /Subsystem/Parasitic Torques/Parasitic AZ ==
  MotTo : Inport
  MotPos : Inport  Port=2
  Cogging : Lookup_n-D  NumberOfTableDimensions=1  LookupTableObject=F_ripple  BreakpointsForDimension1=Pos  Table=Amp_Cog  InternalRulePriority=Speed  RndMeth=Simplest
  Constant : Constant  Value=0.1869
  Divide : Product  Inputs=**
  EMF Distortion : Lookup_n-D  NumberOfTableDimensions=1  LookupTableObject=F_ripple  BreakpointsForDimension1=Pos  Table=Amp_EMF  InternalRulePriority=Speed  RndMeth=Simplest
  Gain : Gain  Gain=1/R
  Gain1 : Gain  Gain=1/250
  Gain2 : Gain  Gain=1/N_Segm
  Mod : Math  Operator=rem  SignedPower=on
  Mod1 : Math  Operator=rem  SignedPower=on
  Radius : Gain  Gain=R
  Sum : Sum  Inputs=|++
  Sum1 : Sum  Inputs=|++
  To : Outport
  wires:
  Radius/1 -> Mod/1  "driven  distance"
  Constant/1 -> Mod1/2, Sum1/2, Mod/2
  MotPos/1 -> Radius/1
  Sum/1 -> To/1
  Cogging/1 -> Sum/2
  MotTo/1 -> Gain/1
  Gain/1 -> Gain1/1  "Force"
  EMF Distortion/1 -> Divide/2
  Divide/1 -> Sum/1
  Gain2/1 -> Divide/1  "I_rms pro Segment"
  Gain1/1 -> Gain2/1  "I_rms"
  Mod/1 -> Sum1/1
  Sum1/1 -> Mod1/1
  Mod1/1 -> EMF Distortion/1, Cogging/1

== system ltao_e2e/Mount_Drv_PDR2021_linear/Parasitic torques model /Subsystem/Parasitic Torques/Parasitic EL ==
  MotTo : Inport
  MotPos : Inport  Port=2
  Cogging : Lookup_n-D  NumberOfTableDimensions=1  LookupTableObject=F_ripple  BreakpointsForDimension1=Pos  Table=Amp_Cog  InternalRulePriority=Speed  RndMeth=Simplest
  Constant : Constant  Value=0.1869
  Divide : Product  Inputs=**
  EMF Distortion : Lookup_n-D  NumberOfTableDimensions=1  LookupTableObject=F_ripple  BreakpointsForDimension1=Pos  Table=Amp_EMF  InternalRulePriority=Speed  RndMeth=Simplest
  Gain : Gain  Gain=1/R
  Gain1 : Gain  Gain=1/250
  Gain2 : Gain  Gain=1/N_Segm
  Mod1 : Math  Operator=rem  SignedPower=on
  Mod2 : Math  Operator=rem  SignedPower=on
  Radius : Gain  Gain=R
  Scope : Scope  Commented=on  NumInputPorts=2
  Sum : Sum  Inputs=|++
  Sum1 : Sum  Inputs=|++
  To : Outport
  wires:
  MotPos/1 -> Radius/1
  Sum/1 -> To/1
  Cogging/1 -> Scope/2, Sum/2
  MotTo/1 -> Gain/1
  Gain/1 -> Gain1/1  "Force"
  EMF Distortion/1 -> Divide/2
  Divide/1 -> Scope/1, Sum/1
  Gain2/1 -> Divide/1  "I_rms pro Segment"
  Gain1/1 -> Gain2/1  "I_rms"
  Sum1/1 -> Mod2/1
  Mod1/1 -> Sum1/1
  Radius/1 -> Mod1/1  "driven distance"
  Constant/1 -> Mod2/2, Sum1/2, Mod1/2
  Mod2/1 -> Cogging/1, EMF Distortion/1

== system ltao_e2e/Mount_Drv_PDR2021_linear/Parasitic torques model /Subsystem/Parasitic Torques/Parasitic GIR ==
  MotTo : Inport
  MotPos : Inport  Port=2
  Cogging : Subsystem
  Emf : Subsystem
  Pretention : Constant  Value=T_pretension
  Product2 : Product  RndMeth=Zero
  Scope : Scope  Commented=on  NumInputPorts=2
  Sign : Signum  ZeroCross=off
  Sum1 : Sum  Inputs=|++
  Sum2 : Sum  Inputs=++|
  To : Outport
  wires:
  Sum2/1 -> To/1
  MotPos/1 -> Cogging/1(Po), Emf/2(Po)
  Cogging/1(T_cog) -> Sum2/2
  Emf/1(T_emf) -> Sum2/1
  Sum1/1 -> Emf/1(To)
  Sign/1 -> Product2/1
  Pretention/1 -> Product2/2
  Product2/1 -> Sum1/2
  MotTo/1 -> Sign/1, Sum1/1

== system ltao_e2e/M2 Control/ASMmodal_Control/ASM_inner_loop_controller_S2/Pre shape + FF terms/Cmd Shaping Filter/If Action Subsystem ==
  In1 : Inport
  In2 : Inport  Port=2
  In3 : Inport  Port=3
  Action Port : ActionPort
  Out1 : Outport  VectorParamsAs1DForOutWhenUnconnected=off
  Out2 : Outport  Port=2  VectorParamsAs1DForOutWhenUnconnected=off
  Out3 : Outport  Port=3  VectorParamsAs1DForOutWhenUnconnected=off
  wires:
  In1/1 -> Out1/1
  In2/1 -> Out2/1
  In3/1 -> Out3/1

== system ltao_e2e/M2 Control/ASMmodal_Control/ASM_inner_loop_controller_S2/Pre shape + FF terms/Cmd Shaping Filter/If Action Subsystem1 ==
  delta : Inport
  Action Port : ActionPort
  Gain : Gain  Gain=0
  Out1 : Outport  VectorParamsAs1DForOutWhenUnconnected=off
  Out2 : Outport  Port=2  VectorParamsAs1DForOutWhenUnconnected=off
  Out3 : Outport  Port=3  VectorParamsAs1DForOutWhenUnconnected=off
  wires:
  delta/1 -> Gain/1, Out3/1
  Gain/1 -> Out1/1, Out2/1

== system ltao_e2e/Mount_Drv_PDR2021_linear/Parasitic torques model /Subsystem/Parasitic Torques/Parasitic GIR/Cogging ==
  Po : Inport
  CogAmp : Constant  Value=cog_amp
  CogSpatFreq : Constant  Value=cog_sfr
  Product1 : Product  RndMeth=Zero
  Product2 : Product  RndMeth=Zero
  Trigonometric Function : Trigonometry
  T_cog : Outport
  wires:
  Product1/1 -> Trigonometric Function/1
  CogSpatFreq/1 -> Product1/2
  CogAmp/1 -> Product2/2
  Trigonometric Function/1 -> Product2/1
  Po/1 -> Product1/1
  Product2/1 -> T_cog/1

== system ltao_e2e/Mount_Drv_PDR2021_linear/Parasitic torques model /Subsystem/Parasitic Torques/Parasitic GIR/Emf ==
  To : Inport
  Po : Inport  Port=2
  EmfAmpFactor : Constant  Value=emf_ampFact
  EmfSpatFreq : Constant  Value=emf_sfr
  Product1 : Product  RndMeth=Zero
  Product2 : Product  Inputs=3  RndMeth=Zero
  Trigonometric Function : Trigonometry
  T_emf : Outport
  wires:
  Product1/1 -> Trigonometric Function/1
  EmfSpatFreq/1 -> Product1/2
  EmfAmpFactor/1 -> Product2/2
  Trigonometric Function/1 -> Product2/1
  Po/1 -> Product1/1
  Product2/1 -> T_emf/1
  To/1 -> Product2/3

== matlab function ltao_e2e/M2 Control/ASMmodal_Control/ASM_inner_loop_controller_S2/Pre shape + FF terms/Command Shaping Filter ==
  data: cmdOld input; cmdSFdd output; cmdSFd output; cmd input; t input; Tcmd input; tSF input; d1SF input; d2SF input; d3SF input; cmdSF output
function [cmdSFdd, cmdSFd, cmdSF] = cmdShFilt(cmdOld, cmd, t, Tcmd, tSF, d1SF, d2SF, d3SF) 
    td = Tcmd;
    nDeltat = floor(t/td);
    tStep = t - td*nDeltat;
    fprintf('tStep:%.3g - nDeltat:%g - td:%.3g\n',tStep,nDeltat,td);
    deltaCmd = cmd - cmdOld;
    if tStep > tSF
        cmdSF = deltaCmd + cmdOld;
        cmdSFd = zeros(size(cmd));
        cmdSFdd = zeros(size(cmd));
    else
        cmdSF = (d1SF/6*tStep^3 + d2SF/12*tStep^4 + d3SF/20*tStep^5)*deltaCmd + cmdOld;
        cmdSFd = (3*d1SF/6*tStep^2 + 4*d2SF/12*tStep^3 + 5*d3SF/20*tStep^4)*deltaCmd;
        cmdSFdd = (6*d1SF/6*tStep + 12*d2SF/12*tStep^2 + 20*d3SF/20*tStep^3)*deltaCmd;
    end
